simulink model "solar_feeder_protection"  (R2025b)
settings: Solver=FixedStepDiscrete  StartTime=0.0  StopTime=1.2  FixedStep=0.001  RelTol=1e-3
settings Model: Creator=Manish  LastModifiedBy=Manish

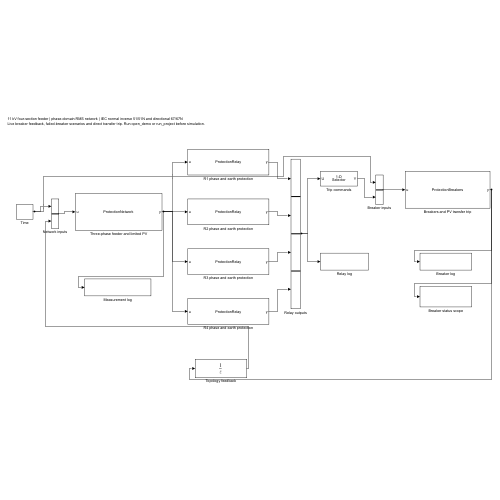
[thumbnail: Simulink's stored preview of the top-level diagram]
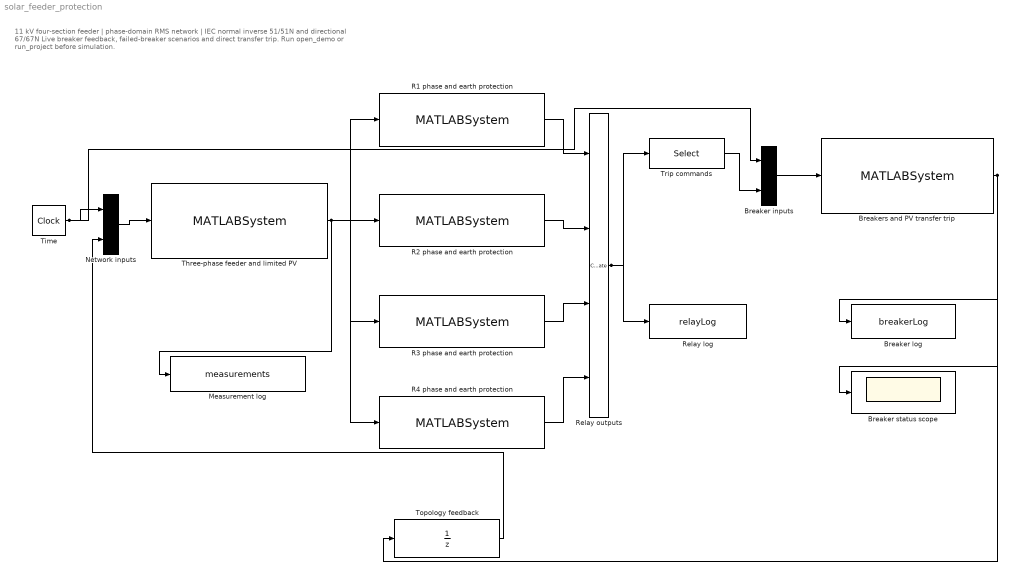
== system solar_feeder_protection ==
  note: 11 kV four-section feeder | phase-domain RMS network | IEC normal inverse 51/51N and directional 67/67N
      | Live breaker feedback, failed-breaker scenarios and direct transfer trip. Run open_demo or run_project before simulation.
  Breaker inputs : Concatenate
  Breaker log : ToWorkspace  VariableName=breakerLog  SaveFormat=Timeseries  SampleTime=-1
  Breaker status scope : Scope
  Breakers and PV transfer trip : MATLABSystem  System=ProtectionBreakers  SimulateUsing=Interpreted execution
      mask Type: ProtectionBreakers
  Measurement log : ToWorkspace  VariableName=measurements  SaveFormat=Timeseries  SampleTime=-1
  Network inputs : Concatenate
  R1 phase and earth protection : MATLABSystem  System=ProtectionRelay  RelayIndex=1  SimulateUsing=Interpreted execution
      mask Type: ProtectionRelay
  R2 phase and earth protection : MATLABSystem  System=ProtectionRelay  RelayIndex=2  SimulateUsing=Interpreted execution
      mask Type: ProtectionRelay
  R3 phase and earth protection : MATLABSystem  System=ProtectionRelay  RelayIndex=3  SimulateUsing=Interpreted execution
      mask Type: ProtectionRelay
  R4 phase and earth protection : MATLABSystem  System=ProtectionRelay  RelayIndex=4  SimulateUsing=Interpreted execution
      mask Type: ProtectionRelay
  Relay log : ToWorkspace  VariableName=relayLog  SaveFormat=Timeseries  SampleTime=-1
  Relay outputs : Concatenate  NumInputs=4
  Three-phase feeder and limited PV : MATLABSystem  System=ProtectionNetwork  SimulateUsing=Interpreted execution
      mask Type: ProtectionNetwork
  Time : DigitalClock  SampleTime=0.001
  Topology feedback : UnitDelay  InitialCondition=ones(1,5)  SampleTime=0.001  HasFrameUpgradeWarning=on
  Trip commands : Selector  InputPortWidth=20  IndexOptions=Index vector (dialog)  Indices=[1 6 11 16]  OutputSizes=1
  wires:
  Three-phase feeder and limited PV/1 -> R1 phase and earth protection/1, R2 phase and earth protection/1, R3 phase and earth protection/1, R4 phase and earth protection/1, Measurement log/1
  R1 phase and earth protection/1 -> Relay outputs/1
  R2 phase and earth protection/1 -> Relay outputs/2
  R3 phase and earth protection/1 -> Relay outputs/3
  R4 phase and earth protection/1 -> Relay outputs/4
  Time/1 -> Network inputs/1, Breaker inputs/1
  Topology feedback/1 -> Network inputs/2
  Network inputs/1 -> Three-phase feeder and limited PV/1
  Relay outputs/1 -> Trip commands/1, Relay log/1
  Trip commands/1 -> Breaker inputs/2
  Breaker inputs/1 -> Breakers and PV transfer trip/1
  Breakers and PV transfer trip/1 -> Topology feedback/1, Breaker log/1, Breaker status scope/1
